simulink model "Roadsense_RoadRunnerIntegration"  (R2025b)
settings: Solver=FixedStepDiscrete  StartTime=0.0  StopTime=inf  FixedStep=RsTsBase  RelTol=1e-3
model workspace (MAT data in the model file):
  RsRoadRunnerScenarioID = 1
undefined symbols (not defined in the file or in its folder): Defined, Ego, Lane, RsTsControl, RsTsScenario, User
libraries: roadrunnerscenario x3
settings Model: DataDictionary=Roadsense_Data.sldd  Creator=ragur  LastModifiedBy=ragur

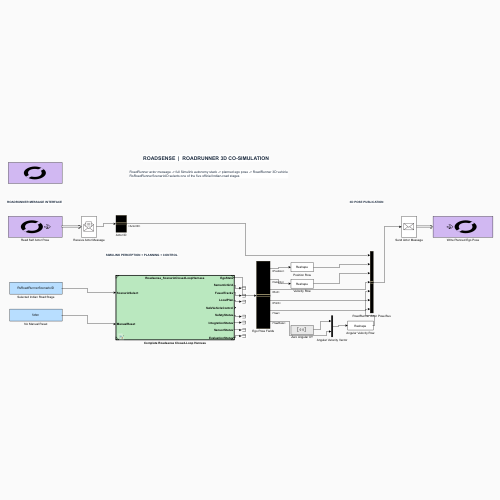
[thumbnail: Simulink's stored preview of the top-level diagram]
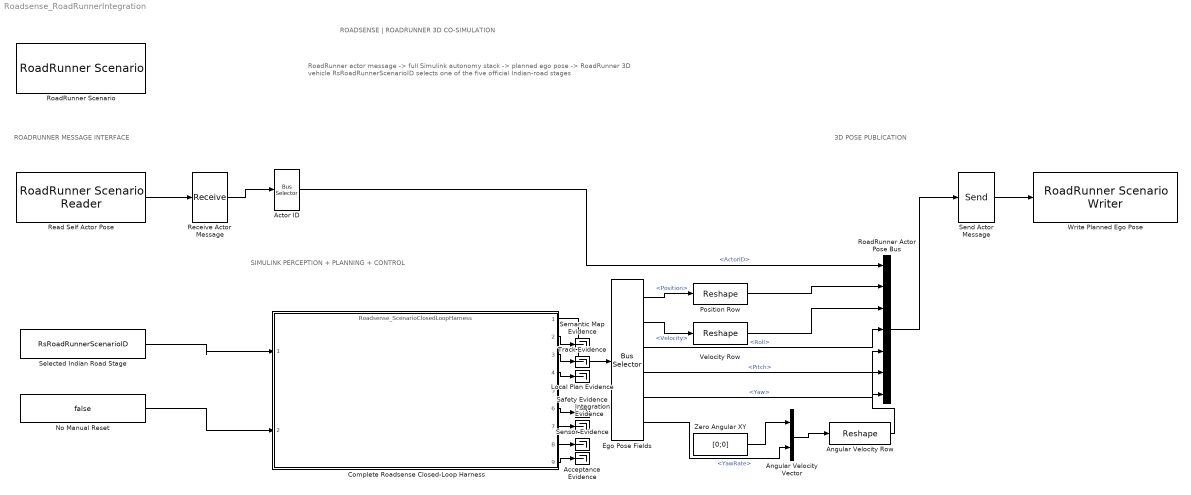
== system Roadsense_RoadRunnerIntegration ==
  note: ROADSENSE | ROADRUNNER 3D CO-SIMULATION
  note: RoadRunner actor message -> full Simulink autonomy stack -> planned ego pose -> RoadRunner 3D vehicle
      | RsRoadRunnerScenarioID selects one of the five official Indian-road stages
  note: ROADRUNNER MESSAGE INTERFACE
  note: SIMULINK PERCEPTION + PLANNING + CONTROL
  note: 3D POSE PUBLICATION
  Acceptance Evidence : Terminator
  Actor ID : BusSelector  OutputSignals=ActorID
  Angular Velocity Row : Reshape  OutputDimensionality=Customize  OutputDimensions=[1 3]
  Angular Velocity Vector : Mux  Inputs=2
  Complete Roadsense Closed-Loop Harness : ModelReference  ModelNameDialog=Roadsense_ScenarioClosedLoopHarness  SimulationMode=Normal  ModelReferenceVersion=1.1
  Ego Pose Fields : BusSelector  OutputSignals=Position,Velocity,Roll,Pitch,Yaw,YawRate
  Integration Evidence : Terminator
  Local Plan Evidence : Terminator
  No Manual Reset : Constant  Value=false  OutDataTypeStr=boolean  SampleTime=RsTsControl
  Position Row : Reshape  OutputDimensionality=Customize  OutputDimensions=[1 3]
  Read Self Actor Pose : roadrunnerscenario/RoadRunner Scenario Reader  TopicCategory=Actor  ActorCategory=All Types  ActionType=Path Following  EventType=User-Defined  TopicType=Actor Pose (Driving Scenario compatible)  VehicleType=Vehicle Specifications  TrafficSignalType=Traffic Signal Specifications  TrafficSignalControllerType=Traffic Signal Controller Specifications  UserDefinedAction=Action1  UserDefinedEvent=Event1  Filter=Self  AdditionalRelationship=None  SensorTopic=Target Poses  LaneBoundaryOutputTopic=Ego-Lane  SensorID=1  SampleTime=RsTsControl
  Receive Actor Message : Receive  InputPortMessageModes=m  UseInternalQueue=off  QueueOverwriting=on  QueueLength=1  QueueType=LIFO  SampleTime=RsTsControl
  RoadRunner Actor Pose Bus : BusCreator  Inputs=7  OutDataTypeStr=Bus: BusActorPose  NonVirtualBus=on
  RoadRunner Scenario : roadrunnerscenario/RoadRunner Scenario  UserDefinedActions={}  UserDefinedEvents={}  PathPoints=500
  Safety Evidence : Terminator
  Selected Indian Road Stage : Constant  Value=RsRoadRunnerScenarioID  OutDataTypeStr=uint8  SampleTime=RsTsScenario
  Semantic Map Evidence : Terminator
  Send Actor Message : Send  OutputPortMessageModes=m
  Sensor Evidence : Terminator
  Track Evidence : Terminator
  Velocity Row : Reshape  OutputDimensionality=Customize  OutputDimensions=[1 3]
  Write Planned Ego Pose : roadrunnerscenario/RoadRunner Scenario Writer  TopicCategory=Actor  ActorCategory=All Types  EventType=Action Complete  UserDefinedEvent=Event1  VehicleType=Vehicle Pose  TopicType=Actor Pose (Driving Scenario compatible)
  Zero Angular XY : Constant  Value=[0;0]  OutDataTypeStr=double
  wires:
  Read Self Actor Pose/1 -> Receive Actor Message/1
  Receive Actor Message/1 -> Actor ID/1
  Selected Indian Road Stage/1 -> Complete Roadsense Closed-Loop Harness/1
  No Manual Reset/1 -> Complete Roadsense Closed-Loop Harness/2
  Complete Roadsense Closed-Loop Harness/1 -> Ego Pose Fields/1
  Ego Pose Fields/1 -> Position Row/1  "<Position>"
  Ego Pose Fields/2 -> Velocity Row/1  "<Velocity>"
  Zero Angular XY/1 -> Angular Velocity Vector/1
  Ego Pose Fields/6 -> Angular Velocity Vector/2  "<YawRate>"
  Angular Velocity Vector/1 -> Angular Velocity Row/1
  Actor ID/1 -> RoadRunner Actor Pose Bus/1  "<ActorID>"
  Position Row/1 -> RoadRunner Actor Pose Bus/2
  Velocity Row/1 -> RoadRunner Actor Pose Bus/3
  Ego Pose Fields/3 -> RoadRunner Actor Pose Bus/4  "<Roll>"
  Ego Pose Fields/4 -> RoadRunner Actor Pose Bus/5  "<Pitch>"
  Ego Pose Fields/5 -> RoadRunner Actor Pose Bus/6  "<Yaw>"
  Angular Velocity Row/1 -> RoadRunner Actor Pose Bus/7
  RoadRunner Actor Pose Bus/1 -> Send Actor Message/1
  Send Actor Message/1 -> Write Planned Ego Pose/1
  Complete Roadsense Closed-Loop Harness/2 -> Semantic Map Evidence/1
  Complete Roadsense Closed-Loop Harness/3 -> Track Evidence/1
  Complete Roadsense Closed-Loop Harness/4 -> Local Plan Evidence/1
  Complete Roadsense Closed-Loop Harness/6 -> Safety Evidence/1
  Complete Roadsense Closed-Loop Harness/7 -> Integration Evidence/1
  Complete Roadsense Closed-Loop Harness/8 -> Sensor Evidence/1
  Complete Roadsense Closed-Loop Harness/9 -> Acceptance Evidence/1
